simulink model "EV_Model_acc"  (R2024b)
settings: Solver=ode23tb  StartTime=0  StopTime=195  RelTol=1e-3
undefined symbols (not defined in the file): Battery, BattSocInit, DiscIntNeverNeededParam, disk_abore, MotSpd, MotTrq, mu_kinetic, Ndiff, Np_Module, Ns_Module, num_pads, NumModules, RegenBrkCutOff, RegenBrkSpd_bpt, Rm
libraries: autolibshared x6, autolibsharedcoupling x3, simulink x3, mpcadaslib x1, autolibdatasheetbattery x1, autolibmappedmotor x1, autolibshareddiff x1, SignalEditorBlockLib x1
(part 3 of 3)

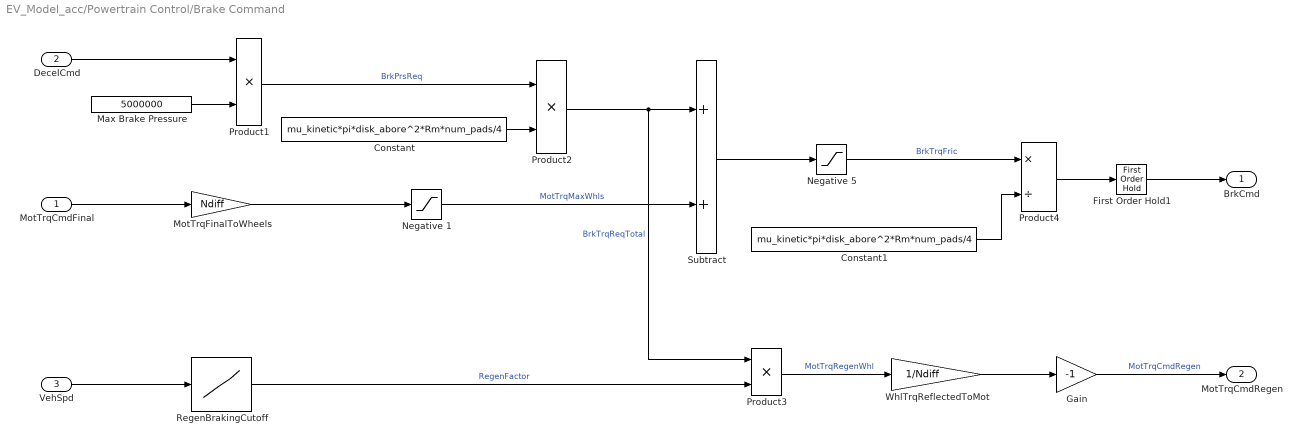
== system EV_Model_acc/Powertrain Control/Brake Command ==
  MotTrqCmdFinal : Inport
  "DecelCmd " : Inport  Port=2
  VehSpd : Inport  Port=3
  Constant : Constant  Value=mu_kinetic*pi*disk_abore^2*Rm*num_pads/4
  Constant1 : Constant  Value=mu_kinetic*pi*disk_abore^2*Rm*num_pads/4
  First Order Hold1 : FirstOrderHold  ErrorTolerance=0.1  AllowContinuousInput=on
  Gain : Gain  Gain=-1
  Max Brake Pressure : Constant  Value=5000000
  MotTrqFinalToWheels : Gain  Gain=Ndiff
  Negative 1 : Saturate  UpperLimit=0  LowerLimit=-inf
  Negative 5 : Saturate  UpperLimit=inf  LowerLimit=0  ZeroCross=off
  Product1 : Product
  Product2 : Product
  Product3 : Product
  Product4 : Product  Inputs=*/
  RegenBrakingCutoff : Lookup_n-D  NumberOfTableDimensions=1  BreakpointsForDimension1=RegenBrkSpd_bpt  Table=RegenBrkCutOff  ExtrapMethod=Clip  UseLastTableValue=on  InternalRulePriority=Speed  RndMeth=Simplest
  Subtract : Sum
  WhlTrqReflectedToMot : Gain  Gain=1/Ndiff
  " BrkCmd" : Outport  VectorParamsAs1DForOutWhenUnconnected=off
  " MotTrqCmdRegen" : Outport  Port=2  VectorParamsAs1DForOutWhenUnconnected=off
  wires:
  Product4/1 -> First Order Hold1/1
  Constant1/1 -> Product4/2
  Constant/1 -> Product2/2
  Product2/1 -> Product3/1, Subtract/1  "BrkTrqReqTotal"
  Subtract/1 -> Negative 5/1
  Negative 5/1 -> Product4/1  "BrkTrqFric"
  MotTrqCmdFinal/1 -> MotTrqFinalToWheels/1
  Negative 1/1 -> Subtract/2  "MotTrqMaxWhls"
  MotTrqFinalToWheels/1 -> Negative 1/1
  Gain/1 -> " MotTrqCmdRegen"/1  "MotTrqCmdRegen"
  WhlTrqReflectedToMot/1 -> Gain/1
  RegenBrakingCutoff/1 -> Product3/2  "RegenFactor"
  Product3/1 -> WhlTrqReflectedToMot/1  "MotTrqRegenWhl"
  VehSpd/1 -> RegenBrakingCutoff/1
  First Order Hold1/1 -> " BrkCmd"/1
  "DecelCmd "/1 -> Product1/1
  Max Brake Pressure/1 -> Product1/2
  Product1/1 -> Product2/1  "BrkPrsReq"

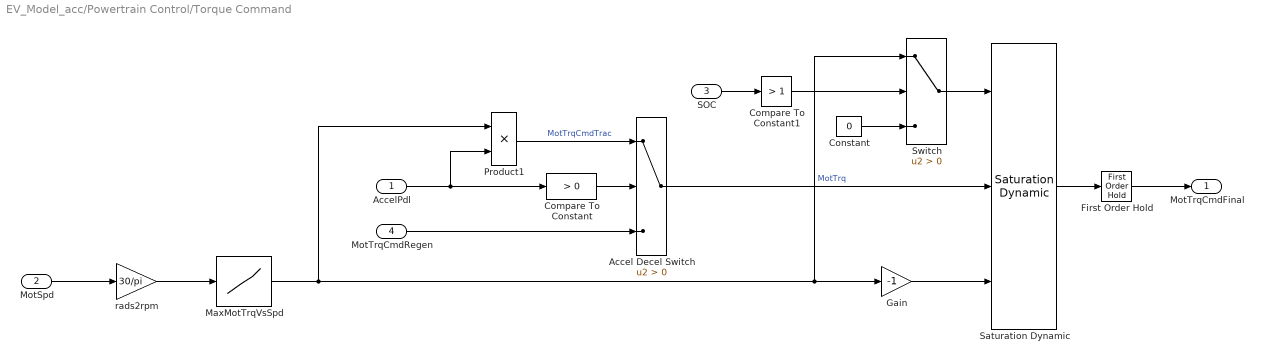
== system EV_Model_acc/Powertrain Control/Torque Command ==
  AccelPdl : Inport
  MotSpd : Inport  Port=2
  SOC : Inport  Port=3
  MotTrqCmdRegen : Inport  Port=4
  Accel Decel Switch : Switch  Criteria=u2 > Threshold  SaturateOnIntegerOverflow=off  InputSameDT=off
  Compare To Constant : simulink/Logic and Bit Operations/Compare To Constant  relop=>  const=0  OutDataTypeStr=boolean
  Compare To Constant1 : simulink/Logic and Bit Operations/Compare To Constant  relop=>  const=1  OutDataTypeStr=boolean
  Constant : Constant  Value=0
  First Order Hold : FirstOrderHold  ErrorTolerance=0.1  AllowContinuousInput=on
  Gain : Gain  Gain=-1
  MaxMotTrqVsSpd : Lookup_n-D  NumberOfTableDimensions=1  BreakpointsForDimension1=MotSpd  Table=MotTrq  ExtrapMethod=Clip  UseLastTableValue=on  InternalRulePriority=Speed  OutDataTypeStr=Inherit: Inherit from 'Table data'  RndMeth=Simplest
  Product1 : Product
  Saturation Dynamic : simulink/Discontinuities/Saturation Dynamic  OutMin=[]  OutMax=[]  OutDataTypeStr=Inherit: Same as second input  OutDataType=fixdt(1, 16)  OutScaling=2^-10  DoSatur=off
  Switch : Switch  Criteria=u2 > Threshold  SaturateOnIntegerOverflow=off  InputSameDT=off
  rads2rpm : Gain  Gain=30/pi
  MotTrqCmdFinal : Outport  VectorParamsAs1DForOutWhenUnconnected=off
  wires:
  Compare To Constant/1 -> Accel Decel Switch/2
  MotTrqCmdRegen/1 -> Accel Decel Switch/3
  Accel Decel Switch/1 -> Saturation Dynamic/2  "MotTrq"
  MotSpd/1 -> rads2rpm/1
  Switch/1 -> Saturation Dynamic/1
  SOC/1 -> Compare To Constant1/1
  Constant/1 -> Switch/3
  Saturation Dynamic/1 -> First Order Hold/1
  Gain/1 -> Saturation Dynamic/3
  Compare To Constant1/1 -> Switch/2
  rads2rpm/1 -> MaxMotTrqVsSpd/1
  Product1/1 -> Accel Decel Switch/1  "MotTrqCmdTrac"
  AccelPdl/1 -> Product1/2, Compare To Constant/1
  MaxMotTrqVsSpd/1 -> Switch/1, Gain/1, Product1/1
  First Order Hold/1 -> MotTrqCmdFinal/1

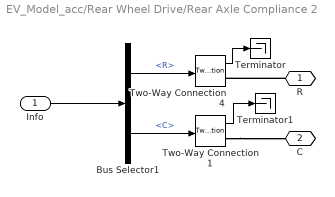
== system EV_Model_acc/Rear Wheel Drive/Rear Axle Compliance 2 ==
  Info : Inport
  Bus Selector1 : BusSelector  OutputSignals=Trq.R,Trq.C
  Terminator : Terminator
  Terminator1 : Terminator
  Two-Way Connection1 : TwoWayConnection
  Two-Way Connection4 : TwoWayConnection
  R : PMIOPort  Side=Left
  C : PMIOPort  Port=2  Side=Right
  wires:
  Two-Way Connection4/1 -> Terminator/1
  Info/1 -> Bus Selector1/1
  Two-Way Connection1/1 -> Terminator1/1
  Bus Selector1/1 -> Two-Way Connection4/1  "<R>"
  Bus Selector1/2 -> Two-Way Connection1/1  "<C>"
  connections:
  R/RConn1 -- Two-Way Connection4/RConn1
  Two-Way Connection1/RConn1 -- C/RConn1

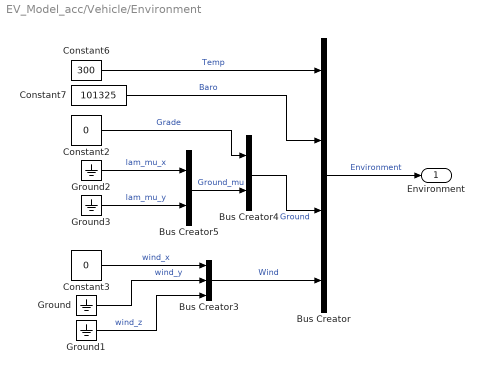
== system EV_Model_acc/Vehicle/Environment ==
  Bus Creator : BusCreator  Inputs=4
  Bus Creator3 : BusCreator  Inputs=3
  Bus Creator4 : BusCreator  Inputs=2
  Bus Creator5 : BusCreator  Inputs=2
  Constant2 : Constant  Value=0
  Constant3 : Constant  Value=0
  Constant6 : Constant  Value=300
  Constant7 : Constant  Value=101325
  Ground{,1..3} (4 alike) : Ground
  Environment : Outport  VectorParamsAs1DForOutWhenUnconnected=off
  wires:
  Constant7/1 -> Bus Creator/2  "Baro"
  Bus Creator/1 -> Environment/1  "Environment"
  Constant2/1 -> Bus Creator4/1  "Grade"
  Constant6/1 -> Bus Creator/1  "Temp"
  Ground1/1 -> Bus Creator3/3  "wind_z"
  Ground/1 -> Bus Creator3/2  "wind_y"
  Constant3/1 -> Bus Creator3/1  "wind_x"
  Bus Creator3/1 -> Bus Creator/4  "Wind"
  Bus Creator4/1 -> Bus Creator/3  "Ground"
  Bus Creator5/1 -> Bus Creator4/2  "Ground_mu"
  Ground3/1 -> Bus Creator5/2  "lam_mu_y"
  Ground2/1 -> Bus Creator5/1  "lam_mu_x"

== matlab function EV_Model_acc/MATLAB Function ==
  data: a_desired input; AccelPID_In output; BrakePID_In output
function [AccelPID_In, BrakePID_In] = processACC(a_desired)
% Split ACC command into positive (acceleration) and negative (braking)

if a_desired >= 0
    AccelPID_In = a_desired;      % Positive accel → Accel PID
    BrakePID_In = 0;
else
    AccelPID_In = 0;
    BrakePID_In = abs(a_desired); % Negative accel → Brake PID
end
